simulink model "Arm_core_design_block"  (R2021a)
settings: Solver=VariableStepAuto  StartTime=0.0  StopTime=600  RelTol=1e-3
undefined symbols (not defined in the file or in its folder): AXI4, Lite
libraries: hdlBasic x979, xbsIndex_r4 x1
(part 1 of 7)
settings Model: Creator=jag33  LastModifiedBy=jag33

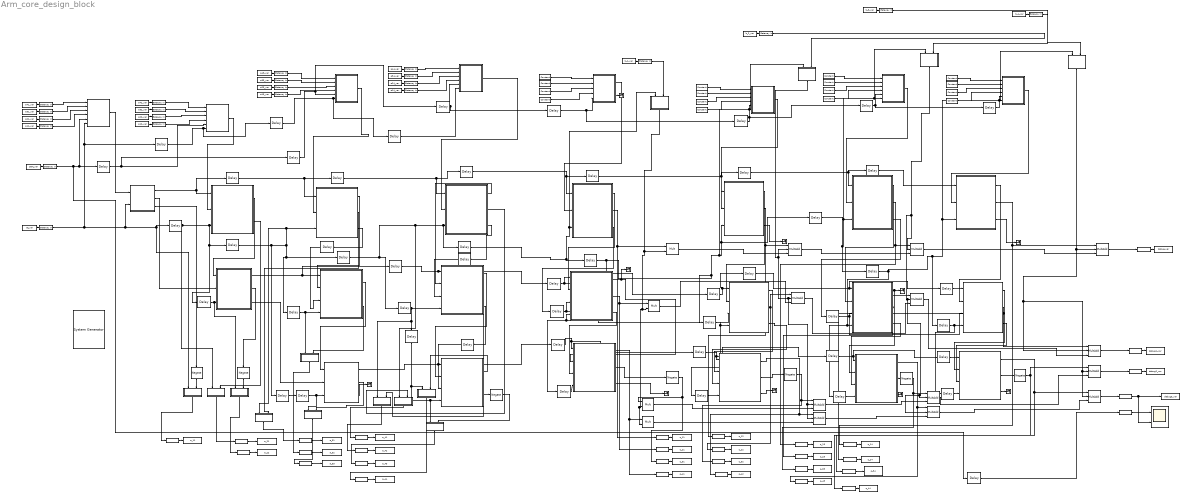
== system Arm_core_design_block ==
  " System Generator" : xbsIndex_r4/ System Generator  Tag=genX  xilinxfamily=zynq  part=xc7z020  speed=-1  package=clg484  synthesis_tool=Vivado  clock_wrapper=Clock Enables  directory=./../../../netlist_proj6_test6  proj_type=Vivado  Synth_file=Vivado Synthesis Defaults  Impl_file=Vivado Implementation Defaults  testbench=off  simulink_period=1  sysclk_period=10  dcm_input_clock_period=10  incr_netlist=off  trim_vbits=Everywhere in SubSystem  dbl_ovrd=According to Block Masks  core_generation=According to Block Masks  run_coregen=off  deprecated_control=off  eval_field=0  block_type=sysgen
  Constant{1..3,6..9,11..14,16} (12 alike) : hdlBasic/Constant  const=0  gui_display_data_type=Fixed-point  arith_type=Signed (2's comp)  n_bits=16  bin_pt=13  preci_type=Single  exp_width=8  frac_width=24  explicit_period=off  period=1  XmcBlockStatus=1  maskContainerNames=tabcontainer1  block_type=constant  block_config=sysgen:Constant_config
  Constant{4..5,10,15} (4 alike) : hdlBasic/Constant  const=1  gui_display_data_type=Fixed-point  arith_type=Signed (2's comp)  n_bits=16  bin_pt=13  preci_type=Single  exp_width=8  frac_width=24  explicit_period=off  period=1  XmcBlockStatus=1  maskContainerNames=tabcontainer1  block_type=constant  block_config=sysgen:Constant_config
  Delay : hdlBasic/Delay  rst=off  en=off  latency=330  reg_retiming=off  XmcBlockStatus=1  maskContainerNames=group1  block_type=delay  block_config=sysgen:Delay_config
  Delay{1..2,6,21,32} (5 alike) : hdlBasic/Delay  rst=off  en=off  latency=25  reg_retiming=off  XmcBlockStatus=1  maskContainerNames=group1  block_type=delay  block_config=sysgen:Delay_config
  Delay{3..5,7..20,22..31,33..49} (44 alike) : hdlBasic/Delay  rst=off  en=off  latency=24  reg_retiming=off  XmcBlockStatus=1  maskContainerNames=group1  block_type=delay  block_config=sysgen:Delay_config
  From Wor43pace1 : FromWorkspace  VariableName=a34_var
  From Work3pace19 : FromWorkspace  VariableName=a33_var
  From Workspace1 : FromWorkspace  VariableName=b_1_var
  From Workspace10 : FromWorkspace  VariableName=a11_var
  From Workspace11 : FromWorkspace  VariableName=a21_var
  From Workspace12 : FromWorkspace  VariableName=a31_var
  From Workspace13 : FromWorkspace  VariableName=a41_var
  From Workspace14 : FromWorkspace  VariableName=a12_var
  From Workspace15 : FromWorkspace  VariableName=a22_var
  From Workspace16 : FromWorkspace  VariableName=a32_var
  From Workspace17 : FromWorkspace  VariableName=a42_var
  From Workspace18 : FromWorkspace  VariableName=a23_var
  From Workspace19 : FromWorkspace  VariableName=a44_var
  From Workspace2 : FromWorkspace  VariableName=rst_var
  From Workspace20 : FromWorkspace  VariableName=a43_var
  From Workspace21 : FromWorkspace  VariableName=a14_var
  From Workspace3 : FromWorkspace  VariableName=start_var
  From Workspace4 : FromWorkspace  VariableName=a13_var
  From Workspace5 : FromWorkspace  VariableName=a24_var
  From Workspace6 : FromWorkspace  VariableName=b_2_var
  From Workspace7 : FromWorkspace  VariableName=b_3_var
  From Workspace8 : FromWorkspace  VariableName=b_4_var
  Mult : hdlBasic/Mult  precision=Full  arith_type="Signed  (2's comp)"  n_bits=16  bin_pt=13  quantization=Truncate  overflow=Wrap  en=off  latency=3  use_behavioral_HDL=off  opt=Speed  use_embedded=on  optimum_pipeline=off  pipeline=on  use_rpm=on  placement_style=Triangular  XmcBlockStatus=1  maskContainerNames=group1  block_type=mult  block_config=sysgen:Mult_config
  Mult1 : hdlBasic/Mult  precision=Full  arith_type="Signed  (2's comp)"  n_bits=16  bin_pt=13  quantization=Truncate  overflow=Wrap  en=off  latency=3  use_behavioral_HDL=off  opt=Speed  use_embedded=on  optimum_pipeline=off  pipeline=on  use_rpm=on  placement_style=Triangular  XmcBlockStatus=1  maskContainerNames=group1  block_type=mult  block_config=sysgen:Mult_config
  Mult2 : hdlBasic/Mult  precision=Full  arith_type="Signed  (2's comp)"  n_bits=16  bin_pt=13  quantization=Truncate  overflow=Wrap  en=off  latency=3  use_behavioral_HDL=off  opt=Speed  use_embedded=on  optimum_pipeline=off  pipeline=on  use_rpm=on  placement_style=Triangular  XmcBlockStatus=1  maskContainerNames=group1  block_type=mult  block_config=sysgen:Mult_config
  Mult3 : hdlBasic/Mult  precision=Full  arith_type="Signed  (2's comp)"  n_bits=16  bin_pt=14  quantization=Truncate  overflow=Wrap  en=off  latency=3  use_behavioral_HDL=off  opt=Speed  use_embedded=on  optimum_pipeline=off  pipeline=on  use_rpm=on  placement_style=Triangular  XmcBlockStatus=1  maskContainerNames=group1  block_type=mult  block_config=sysgen:Mult_config
  MultAdd : hdlBasic/MultAdd  mode=Addition  en=off  latency=0  precision=Full  arith_type="Signed  (2's comp)"  n_bits=16  bin_pt=13  XmcBlockStatus=1  maskContainerNames=tabcontainer1  block_type=multadd  block_config=sysgen:MultAdd_config
  MultAdd{1,7..10} (5 alike) : hdlBasic/MultAdd  mode=Addition  en=off  latency=0  precision=Full  arith_type=Unsigned  n_bits=16  bin_pt=14  XmcBlockStatus=1  maskContainerNames=tabcontainer1  block_type=multadd  block_config=sysgen:MultAdd_config
  MultAdd11 : hdlBasic/MultAdd  mode=Addition  en=off  latency=0  precision=User Defined  arith_type="Signed  (2's comp)"  n_bits=16  bin_pt=13  XmcBlockStatus=1  maskContainerNames=tabcontainer1  block_type=multadd  block_config=sysgen:MultAdd_config
  MultAdd2 : hdlBasic/MultAdd  mode=Addition  en=off  latency=0  precision=User Defined  arith_type="Signed  (2's comp)"  n_bits=16  bin_pt=13  XmcBlockStatus=1  maskContainerNames=tabcontainer1  block_type=multadd  block_config=sysgen:MultAdd_config
  MultAdd3 : hdlBasic/MultAdd  mode=Addition  en=off  latency=0  precision=Full  arith_type=Unsigned  n_bits=16  bin_pt=13  XmcBlockStatus=1  maskContainerNames=tabcontainer1  block_type=multadd  block_config=sysgen:MultAdd_config
  MultAdd4 : hdlBasic/MultAdd  mode=Addition  en=off  latency=0  precision=Full  arith_type=Unsigned  n_bits=16  bin_pt=13  XmcBlockStatus=1  maskContainerNames=tabcontainer1  block_type=multadd  block_config=sysgen:MultAdd_config
  MultAdd5 : hdlBasic/MultAdd  mode=Addition  en=off  latency=0  precision=User Defined  arith_type="Signed  (2's comp)"  n_bits=16  bin_pt=13  XmcBlockStatus=1  maskContainerNames=tabcontainer1  block_type=multadd  block_config=sysgen:MultAdd_config
  MultAdd6 : hdlBasic/MultAdd  mode=Addition  en=off  latency=0  precision=User Defined  arith_type=Unsigned  n_bits=16  bin_pt=13  XmcBlockStatus=1  maskContainerNames=tabcontainer1  block_type=multadd  block_config=sysgen:MultAdd_config
  Negate{1..4,6,8,10} (7 alike) : hdlBasic/Negate  precision=User Defined  arith_type="Signed  (2's comp)"  n_bits=16  bin_pt=13  quantization=Truncate  overflow=Wrap  en=off  latency=0  XmcBlockStatus=1  maskContainerNames=tabcontainer1  block_type=negate  block_config=sysgen:Negate_config
  Scope : Scope  NumInputPorts=2
  Subsystem : Subsystem
  Subsystem1 : Subsystem
  Subsystem10 : Subsystem
  Subsystem11 : Subsystem
  Subsystem13 : Subsystem
  Subsystem14 : Subsystem
  Subsystem15 : Subsystem
  Subsystem16 : Subsystem
  Subsystem17 : Subsystem
  Subsystem18 : Subsystem
  Subsystem19 : Subsystem
  Subsystem2 : Subsystem
  Subsystem20 : Subsystem
  Subsystem21 : Subsystem
  Subsystem22 : Subsystem
  Subsystem3 : Subsystem
  Subsystem4 : Subsystem
  Subsystem5 : Subsystem
  Subsystem6 : Subsystem
  Subsystem7 : Subsystem
  Subsystem8 : Subsystem
  Subsystem9 : Subsystem
  Terminator{,1..8,13} (10 alike) : Terminator
  To Workspace1 : ToWorkspace  VariableName=q_11  SaveFormat=Timeseries  SampleTime=-1
  To Workspace10 : ToWorkspace  VariableName=a_41  SaveFormat=Timeseries  SampleTime=-1
  To Workspace11 : ToWorkspace  VariableName=a_44  SaveFormat=Timeseries  SampleTime=-1
  To Workspace12 : ToWorkspace  VariableName=a_42  SaveFormat=Timeseries  SampleTime=-1
  To Workspace13 : ToWorkspace  VariableName=a_43  SaveFormat=Timeseries  SampleTime=-1
  To Workspace14 : ToWorkspace  VariableName=q_21  SaveFormat=Timeseries  SampleTime=-1
  To Workspace15 : ToWorkspace  VariableName=q_31  SaveFormat=Timeseries  SampleTime=-1
  To Workspace16 : ToWorkspace  VariableName=q_41  SaveFormat=Timeseries  SampleTime=-1
  To Workspace17 : ToWorkspace  VariableName=q_42  SaveFormat=Timeseries  SampleTime=-1
  To Workspace18 : ToWorkspace  VariableName=q_32  SaveFormat=Timeseries  SampleTime=-1
  To Workspace19 : ToWorkspace  VariableName=q_13  SaveFormat=Timeseries  SampleTime=-1
  To Workspace2 : ToWorkspace  VariableName=a_22  SaveFormat=Timeseries  SampleTime=-1
  To Workspace20 : ToWorkspace  VariableName=q_23  SaveFormat=Timeseries  SampleTime=-1
  To Workspace21 : ToWorkspace  VariableName=q_33  SaveFormat=Timeseries  SampleTime=-1
  To Workspace22 : ToWorkspace  VariableName=q_43  SaveFormat=Timeseries  SampleTime=-1
  To Workspace23 : ToWorkspace  VariableName=q_44  SaveFormat=Timeseries  SampleTime=-1
  To Workspace24 : ToWorkspace  VariableName=q_24  SaveFormat=Timeseries  SampleTime=-1
  To Workspace25 : ToWorkspace  VariableName=q_14  SaveFormat=Timeseries  SampleTime=-1
  To Workspace26 : ToWorkspace  VariableName=q_34  SaveFormat=Timeseries  SampleTime=-1
  To Workspace27 : ToWorkspace  VariableName=debug_var  SaveFormat=Timeseries  SampleTime=-1
  To Workspace28 : ToWorkspace  VariableName=debug1_var  SaveFormat=Timeseries  SampleTime=-1
  To Workspace29 : ToWorkspace  VariableName=debug2_var  SaveFormat=Timeseries  SampleTime=-1
  To Workspace3 : ToWorkspace  VariableName=a_11  SaveFormat=Timeseries  SampleTime=-1
  To Workspace30 : ToWorkspace  VariableName=debug3_var  SaveFormat=Timeseries  SampleTime=-1
  To Workspace4 : ToWorkspace  VariableName=q_12  SaveFormat=Timeseries  SampleTime=-1
  To Workspace5 : ToWorkspace  VariableName=a_21  SaveFormat=Timeseries  SampleTime=-1
  To Workspace6 : ToWorkspace  VariableName=a_31  SaveFormat=Timeseries  SampleTime=-1
  To Workspace7 : ToWorkspace  VariableName=q_22  SaveFormat=Timeseries  SampleTime=-1
  To Workspace8 : ToWorkspace  VariableName=a_32  SaveFormat=Timeseries  SampleTime=-1
  To Workspace9 : ToWorkspace  VariableName=a_33  SaveFormat=Timeseries  SampleTime=-1
  a11_var : hdlBasic/Gateway In  gui_display_data_type=Fixed-point  arith_type=Signed (2's comp)  n_bits=16  bin_pt=13  preci_type=Single  exp_width=8  frac_width=24  rows=1  columns=1  quantization="Round  (unbiased: +/- Inf)"  overflow=Saturate  period=1  UseAsADC=off  ADCChannel='1'  interface=AXI4-Lite  automatic_assignment=on  address_offset=hex2dec('00')  intf_name=''  intf_description=''  default_value=0  timing_constraint=None  locs_specified=off  LOCs={}  io_standard={}  inherit_from_input=off  hdl_port=on  XmcBlockStatus=1  maskContainerNames=group4  block_type=gatewayin  block_config=sysgen:gateway_in_config  block_width_w=590  block_height_w=620  block_width=640  block_height=850
  a12_var : hdlBasic/Gateway In  gui_display_data_type=Fixed-point  arith_type=Signed (2's comp)  n_bits=16  bin_pt=13  preci_type=Single  exp_width=8  frac_width=24  rows=1  columns=1  quantization="Round  (unbiased: +/- Inf)"  overflow=Saturate  period=1  UseAsADC=off  ADCChannel='1'  interface=AXI4-Lite  automatic_assignment=on  address_offset=hex2dec('00')  intf_name=''  intf_description=''  default_value=0  timing_constraint=None  locs_specified=off  LOCs={}  io_standard={}  inherit_from_input=off  hdl_port=on  XmcBlockStatus=1  maskContainerNames=group4  block_type=gatewayin  block_config=sysgen:gateway_in_config  block_width_w=590  block_height_w=620  block_width=640  block_height=850
  a13_var : hdlBasic/Gateway In  gui_display_data_type=Fixed-point  arith_type=Signed (2's comp)  n_bits=16  bin_pt=13  preci_type=Single  exp_width=8  frac_width=24  rows=1  columns=1  quantization="Round  (unbiased: +/- Inf)"  overflow=Saturate  period=1  UseAsADC=off  ADCChannel='1'  interface=AXI4-Lite  automatic_assignment=on  address_offset=hex2dec('00')  intf_name=''  intf_description=''  default_value=0  timing_constraint=None  locs_specified=off  LOCs={}  io_standard={}  inherit_from_input=off  hdl_port=on  XmcBlockStatus=1  maskContainerNames=group4  block_type=gatewayin  block_config=sysgen:gateway_in_config  block_width_w=590  block_height_w=620  block_width=640  block_height=850
  a14_var : hdlBasic/Gateway In  gui_display_data_type=Fixed-point  arith_type=Signed (2's comp)  n_bits=16  bin_pt=13  preci_type=Single  exp_width=8  frac_width=24  rows=1  columns=1  quantization="Round  (unbiased: +/- Inf)"  overflow=Saturate  period=1  UseAsADC=off  ADCChannel='1'  interface=AXI4-Lite  automatic_assignment=on  address_offset=hex2dec('00')  intf_name=''  intf_description=''  default_value=0  timing_constraint=None  locs_specified=off  LOCs={}  io_standard={}  inherit_from_input=off  hdl_port=on  XmcBlockStatus=1  maskContainerNames=group4  block_type=gatewayin  block_config=sysgen:gateway_in_config  block_width_w=590  block_height_w=620  block_width=640  block_height=850
  a21_var : hdlBasic/Gateway In  gui_display_data_type=Fixed-point  arith_type=Signed (2's comp)  n_bits=16  bin_pt=13  preci_type=Single  exp_width=8  frac_width=24  rows=1  columns=1  quantization="Round  (unbiased: +/- Inf)"  overflow=Saturate  period=1  UseAsADC=off  ADCChannel='1'  interface=AXI4-Lite  automatic_assignment=on  address_offset=hex2dec('00')  intf_name=''  intf_description=''  default_value=0  timing_constraint=None  locs_specified=off  LOCs={}  io_standard={}  inherit_from_input=off  hdl_port=on  XmcBlockStatus=1  maskContainerNames=group4  block_type=gatewayin  block_config=sysgen:gateway_in_config  block_width_w=590  block_height_w=620  block_width=640  block_height=850
  a22_var : hdlBasic/Gateway In  gui_display_data_type=Fixed-point  arith_type=Signed (2's comp)  n_bits=16  bin_pt=13  preci_type=Single  exp_width=8  frac_width=24  rows=1  columns=1  quantization="Round  (unbiased: +/- Inf)"  overflow=Saturate  period=1  UseAsADC=off  ADCChannel='1'  interface=AXI4-Lite  automatic_assignment=on  address_offset=hex2dec('00')  intf_name=''  intf_description=''  default_value=0  timing_constraint=None  locs_specified=off  LOCs={}  io_standard={}  inherit_from_input=off  hdl_port=on  XmcBlockStatus=1  maskContainerNames=group4  block_type=gatewayin  block_config=sysgen:gateway_in_config  block_width_w=590  block_height_w=620  block_width=640  block_height=850
  a23_var : hdlBasic/Gateway In  gui_display_data_type=Fixed-point  arith_type=Signed (2's comp)  n_bits=16  bin_pt=13  preci_type=Single  exp_width=8  frac_width=24  rows=1  columns=1  quantization="Round  (unbiased: +/- Inf)"  overflow=Saturate  period=1  UseAsADC=off  ADCChannel='1'  interface=AXI4-Lite  automatic_assignment=on  address_offset=hex2dec('00')  intf_name=''  intf_description=''  default_value=0  timing_constraint=None  locs_specified=off  LOCs={}  io_standard={}  inherit_from_input=off  hdl_port=on  XmcBlockStatus=1  maskContainerNames=group4  block_type=gatewayin  block_config=sysgen:gateway_in_config  block_width_w=590  block_height_w=620  block_width=640  block_height=850
  a24_var : hdlBasic/Gateway In  gui_display_data_type=Fixed-point  arith_type=Signed (2's comp)  n_bits=16  bin_pt=13  preci_type=Single  exp_width=8  frac_width=24  rows=1  columns=1  quantization="Round  (unbiased: +/- Inf)"  overflow=Saturate  period=1  UseAsADC=off  ADCChannel='1'  interface=AXI4-Lite  automatic_assignment=on  address_offset=hex2dec('00')  intf_name=''  intf_description=''  default_value=0  timing_constraint=None  locs_specified=off  LOCs={}  io_standard={}  inherit_from_input=off  hdl_port=on  XmcBlockStatus=1  maskContainerNames=group4  block_type=gatewayin  block_config=sysgen:gateway_in_config  block_width_w=590  block_height_w=620  block_width=640  block_height=850
  a31_var : hdlBasic/Gateway In  gui_display_data_type=Fixed-point  arith_type=Signed (2's comp)  n_bits=16  bin_pt=13  preci_type=Single  exp_width=8  frac_width=24  rows=1  columns=1  quantization="Round  (unbiased: +/- Inf)"  overflow=Saturate  period=1  UseAsADC=off  ADCChannel='1'  interface=AXI4-Lite  automatic_assignment=on  address_offset=hex2dec('00')  intf_name=''  intf_description=''  default_value=0  timing_constraint=None  locs_specified=off  LOCs={}  io_standard={}  inherit_from_input=off  hdl_port=on  XmcBlockStatus=1  maskContainerNames=group4  block_type=gatewayin  block_config=sysgen:gateway_in_config  block_width_w=590  block_height_w=620  block_width=640  block_height=850
  a32_var : hdlBasic/Gateway In  gui_display_data_type=Fixed-point  arith_type=Signed (2's comp)  n_bits=16  bin_pt=13  preci_type=Single  exp_width=8  frac_width=24  rows=1  columns=1  quantization="Round  (unbiased: +/- Inf)"  overflow=Saturate  period=1  UseAsADC=off  ADCChannel='1'  interface=AXI4-Lite  automatic_assignment=on  address_offset=hex2dec('00')  intf_name=''  intf_description=''  default_value=0  timing_constraint=None  locs_specified=off  LOCs={}  io_standard={}  inherit_from_input=off  hdl_port=on  XmcBlockStatus=1  maskContainerNames=group4  block_type=gatewayin  block_config=sysgen:gateway_in_config  block_width_w=590  block_height_w=620  block_width=640  block_height=850
  a33_var : hdlBasic/Gateway In  gui_display_data_type=Fixed-point  arith_type=Signed (2's comp)  n_bits=16  bin_pt=13  preci_type=Single  exp_width=8  frac_width=24  rows=1  columns=1  quantization="Round  (unbiased: +/- Inf)"  overflow=Saturate  period=1  UseAsADC=off  ADCChannel='1'  interface=AXI4-Lite  automatic_assignment=on  address_offset=hex2dec('00')  intf_name=''  intf_description=''  default_value=0  timing_constraint=None  locs_specified=off  LOCs={}  io_standard={}  inherit_from_input=off  hdl_port=on  XmcBlockStatus=1  maskContainerNames=group4  block_type=gatewayin  block_config=sysgen:gateway_in_config  block_width_w=590  block_height_w=620  block_width=640  block_height=850
  a34_var : hdlBasic/Gateway In  gui_display_data_type=Fixed-point  arith_type=Signed (2's comp)  n_bits=16  bin_pt=13  preci_type=Single  exp_width=8  frac_width=24  rows=1  columns=1  quantization="Round  (unbiased: +/- Inf)"  overflow=Saturate  period=1  UseAsADC=off  ADCChannel='1'  interface=AXI4-Lite  automatic_assignment=on  address_offset=hex2dec('00')  intf_name=''  intf_description=''  default_value=0  timing_constraint=None  locs_specified=off  LOCs={}  io_standard={}  inherit_from_input=off  hdl_port=on  XmcBlockStatus=1  maskContainerNames=group4  block_type=gatewayin  block_config=sysgen:gateway_in_config  block_width_w=590  block_height_w=620  block_width=640  block_height=850
  a41_var : hdlBasic/Gateway In  gui_display_data_type=Fixed-point  arith_type=Signed (2's comp)  n_bits=16  bin_pt=13  preci_type=Single  exp_width=8  frac_width=24  rows=1  columns=1  quantization="Round  (unbiased: +/- Inf)"  overflow=Saturate  period=1  UseAsADC=off  ADCChannel='1'  interface=AXI4-Lite  automatic_assignment=on  address_offset=hex2dec('00')  intf_name=''  intf_description=''  default_value=0  timing_constraint=None  locs_specified=off  LOCs={}  io_standard={}  inherit_from_input=off  hdl_port=on  XmcBlockStatus=1  maskContainerNames=group4  block_type=gatewayin  block_config=sysgen:gateway_in_config  block_width_w=590  block_height_w=620  block_width=640  block_height=850
  a42_var : hdlBasic/Gateway In  gui_display_data_type=Fixed-point  arith_type=Signed (2's comp)  n_bits=16  bin_pt=13  preci_type=Single  exp_width=8  frac_width=24  rows=1  columns=1  quantization="Round  (unbiased: +/- Inf)"  overflow=Saturate  period=1  UseAsADC=off  ADCChannel='1'  interface=AXI4-Lite  automatic_assignment=on  address_offset=hex2dec('00')  intf_name=''  intf_description=''  default_value=0  timing_constraint=None  locs_specified=off  LOCs={}  io_standard={}  inherit_from_input=off  hdl_port=on  XmcBlockStatus=1  maskContainerNames=group4  block_type=gatewayin  block_config=sysgen:gateway_in_config  block_width_w=590  block_height_w=620  block_width=640  block_height=850
  a43_var : hdlBasic/Gateway In  gui_display_data_type=Fixed-point  arith_type=Signed (2's comp)  n_bits=16  bin_pt=13  preci_type=Single  exp_width=8  frac_width=24  rows=1  columns=1  quantization="Round  (unbiased: +/- Inf)"  overflow=Saturate  period=1  UseAsADC=off  ADCChannel='1'  interface=AXI4-Lite  automatic_assignment=on  address_offset=hex2dec('00')  intf_name=''  intf_description=''  default_value=0  timing_constraint=None  locs_specified=off  LOCs={}  io_standard={}  inherit_from_input=off  hdl_port=on  XmcBlockStatus=1  maskContainerNames=group4  block_type=gatewayin  block_config=sysgen:gateway_in_config  block_width_w=590  block_height_w=620  block_width=640  block_height=850
  a44_var : hdlBasic/Gateway In  gui_display_data_type=Fixed-point  arith_type=Signed (2's comp)  n_bits=16  bin_pt=13  preci_type=Single  exp_width=8  frac_width=24  rows=1  columns=1  quantization="Round  (unbiased: +/- Inf)"  overflow=Saturate  period=1  UseAsADC=off  ADCChannel='1'  interface=AXI4-Lite  automatic_assignment=on  address_offset=hex2dec('00')  intf_name=''  intf_description=''  default_value=0  timing_constraint=None  locs_specified=off  LOCs={}  io_standard={}  inherit_from_input=off  hdl_port=on  XmcBlockStatus=1  maskContainerNames=group4  block_type=gatewayin  block_config=sysgen:gateway_in_config  block_width_w=590  block_height_w=620  block_width=640  block_height=850
  arctan1 : Subsystem
  arctan2 : Subsystem
  arctan3 : Subsystem
  b_{1..4} (4 alike) : hdlBasic/Gateway In  gui_display_data_type=Fixed-point  arith_type=Signed (2's comp)  n_bits=16  bin_pt=13  preci_type=Single  exp_width=8  frac_width=24  rows=1  columns=1  quantization="Round  (unbiased: +/- Inf)"  overflow=Saturate  period=1  UseAsADC=off  ADCChannel='1'  interface=AXI4-Lite  automatic_assignment=on  address_offset=hex2dec('00')  intf_name=''  intf_description=''  default_value=0  timing_constraint=None  locs_specified=off  LOCs={}  io_standard={}  inherit_from_input=off  hdl_port=on  XmcBlockStatus=1  maskContainerNames=group4  block_type=gatewayin  block_config=sysgen:gateway_in_config  block_width_w=590  block_height_w=620  block_width=640  block_height=850
  done_var : hdlBasic/Gateway Out  inherit_from_input=off  hdl_port=on  rows=1  columns=1  UseAsDAC=off  DACChannel='1'  interface=AXI4-Lite  automatic_assignment=on  address_offset=hex2dec('00')  intf_name=''  intf_description=''  timing_constraint=None  locs_specified=off  LOCs={}  io_standard={}  XmcBlockStatus=1  maskContainerNames=group4  block_type=gatewayout  block_config=sysgen:gateway_out_config  block_width_w=590  block_height_w=620  block_width=620  block_height=750
  qout_{1..4,11..14,21..24,31..34,41..44} (20 alike) : hdlBasic/Gateway Out  inherit_from_input=off  hdl_port=on  rows=1  columns=1  UseAsDAC=off  DACChannel='1'  interface=AXI4-Lite  automatic_assignment=on  address_offset=hex2dec('00')  intf_name=''  intf_description=''  timing_constraint=None  locs_specified=off  LOCs={}  io_standard={}  XmcBlockStatus=1  maskContainerNames=group4  block_type=gatewayout  block_config=sysgen:gateway_out_config  block_width_w=590  block_height_w=620  block_width=620  block_height=750
  rotation1 : Subsystem
  rotation10 : Subsystem
  rotation11 : Subsystem
  rotation12 : Subsystem
  rotation13 : Subsystem
  rotation14 : Subsystem
  rotation15 : Subsystem
  rotation16 : Subsystem
  rotation17 : Subsystem
  rotation19 : Subsystem
  rotation2 : Subsystem
  rotation3 : Subsystem
  rotation4 : Subsystem
  rotation5 : Subsystem
  rotation6 : Subsystem
  rotation7 : Subsystem
  rotation8 : Subsystem
  rotation9 : Subsystem
  rout_{11,21..22,31..33,41..44} (10 alike) : hdlBasic/Gateway Out  inherit_from_input=off  hdl_port=on  rows=1  columns=1  UseAsDAC=off  DACChannel='1'  interface=AXI4-Lite  automatic_assignment=on  address_offset=hex2dec('00')  intf_name=''  intf_description=''  timing_constraint=None  locs_specified=off  LOCs={}  io_standard={}  XmcBlockStatus=1  maskContainerNames=group4  block_type=gatewayout  block_config=sysgen:gateway_out_config  block_width_w=590  block_height_w=620  block_width=620  block_height=750
  rst_var : hdlBasic/Gateway In  gui_display_data_type=Boolean  arith_type=Boolean  n_bits=16  bin_pt=13  preci_type=Single  exp_width=8  frac_width=24  rows=1  columns=1  quantization="Round  (unbiased: +/- Inf)"  overflow=Saturate  period=1  UseAsADC=off  ADCChannel='1'  interface=AXI4-Lite  automatic_assignment=on  address_offset=hex2dec('00')  intf_name=''  intf_description=''  default_value=0  timing_constraint=None  locs_specified=off  LOCs={}  io_standard={}  inherit_from_input=off  hdl_port=on  XmcBlockStatus=1  maskContainerNames=group4  block_type=gatewayin  block_config=sysgen:gateway_in_config  block_width_w=590  block_height_w=620  block_width=640  block_height=850
  start_var : hdlBasic/Gateway In  gui_display_data_type=Boolean  arith_type=Boolean  n_bits=16  bin_pt=13  preci_type=Single  exp_width=8  frac_width=24  rows=1  columns=1  quantization="Round  (unbiased: +/- Inf)"  overflow=Saturate  period=1  UseAsADC=off  ADCChannel='1'  interface=AXI4-Lite  automatic_assignment=on  address_offset=hex2dec('00')  intf_name=''  intf_description=''  default_value=0  timing_constraint=None  locs_specified=off  LOCs={}  io_standard={}  inherit_from_input=off  hdl_port=on  XmcBlockStatus=1  maskContainerNames=group4  block_type=gatewayin  block_config=sysgen:gateway_in_config  block_width_w=590  block_height_w=620  block_width=640  block_height=850
  wires:
  Subsystem14/1(fifo_out) -> rotation1/2(y_in)
  rotation1/1(s_out) -> arctan2/1(y_in)
  rout_21/1 -> To Workspace5/1  "rout_21"
  rout_11/1 -> To Workspace3/1  "c"
  rotation1/2(c_out1) -> Subsystem1/2(reg_i)
  arctan1/1(out_theta) -> Delay5/1, rotation1/1(Theta_in)
  rout_31/1 -> To Workspace6/1  "out_31"
  rotation2/1(s_out) -> rotation3/2(y_in)
  Subsystem21/1(fifo_out) -> rotation2/2(y_in)
  rout_22/1 -> To Workspace2/1  "out_22"
  arctan1/2(ready) -> arctan2/2(sel)
  arctan2/1(out_theta) -> rotation3/1(Theta_in), Delay4/1
  rotation2/3(sel_out) -> Delay2/1
  Delay2/1 -> rotation3/3(sel_in)
  Delay5/1 -> rotation2/1(Theta_in), Delay3/1
  Delay3/1 -> rotation4/1(Theta_in), Delay7/1
  Subsystem11/1(fifo_out) -> rotation4/2(y_in)
  rotation2/2(c_out1) -> Subsystem3/2(reg_i)
  rout_32/1 -> To Workspace8/1  "out_32"
  arctan2/3(ready) -> arctan3/2(sel)
  rout_33/1 -> To Workspace9/1  "out_33"
  arctan2/2(cos_val) -> Negate3/1
  arctan3/3(ready) -> Terminator/1
  arctan3/1(out_theta) -> Delay22/1, rotation6/1(Theta_in)
  rotation4/3(sel_out) -> Delay1/1
  rotation4/1(s_out) -> rotation5/2(y_in)
  rotation3/1(s_out) -> arctan3/1(y_in)
  rotation3/2(c_out1) -> Subsystem4/2(reg_i)
  rout_41/1 -> To Workspace10/1  "out_41"
  Delay1/1 -> rotation5/3(sel_in)
  Delay4/1 -> Delay20/1, rotation5/1(Theta_in)
  rout_42/1 -> To Workspace12/1  "out_42"
  rotation5/2(c_out1) -> Subsystem7/2(reg_i)
  rotation5/1(s_out) -> rotation6/2(y_in)
  rotation5/3(sel_out) -> Delay6/1
  Delay6/1 -> rotation6/3(sel_in)
  rout_44/1 -> To Workspace11/1  "out_44"
  rout_43/1 -> To Workspace13/1  "out_43"
  Negate2/1 -> Subsystem8/2(reg_i)
  rotation6/2(c_out1) -> Negate2/1
  Subsystem13/1(fifo_out) -> rotation8/2(y_in)
  Delay7/1 -> rotation8/1(Theta_in), Delay19/1
  rotation8/3(sel_out) -> Delay21/1
  qout_11/1 -> To Workspace1/1  "c_r_out"
  rotation8/2(c_out1) -> qout_11/1, Mult/1
  From Workspace2/1 -> rst_var/1
  Delay8/1 -> Delay9/1, Delay12/1, rotation1/3(rst), Subsystem1/1(rst)
  Delay9/1 -> Delay13/1, Delay10/1, rotation2/3(rst), Subsystem3/1(rst), Delay14/1
  Delay12/1 -> Subsystem2/1(rst), arctan2/3(rst)
  Delay13/1 -> Subsystem4/1(rst), rotation3/4(rst)
  Delay14/1 -> Delay15/1
  Delay15/1 -> Subsystem5/1(rst), arctan3/3(rst)
  Delay16/1 -> Subsystem7/1(rst), Delay17/1, rotation5/4(rst)
  Delay17/1 -> Subsystem9/1(rst), rotation6/4(rst), Subsystem8/1(rst)
  Subsystem16/1(fifo_out) -> rotation7/2(y_in)
  Delay19/1 -> rotation7/1(Theta_in), Delay40/1
  rotation7/2(c_out1) -> qout_12/1, MultAdd/1
  rotation7/3(sel_out) -> Terminator4/1
  qout_12/1 -> To Workspace4/1  "c_r_out"
  qout_22/1 -> To Workspace7/1  "c_r_out"
  Delay20/1 -> Delay25/1, rotation9/1(Theta_in)
  rotation8/1(s_out) -> rotation9/2(y_in)
  Delay21/1 -> rotation11/3(sel_in), rotation9/3(sel_in)
  qout_21/1 -> To Workspace14/1  "c_r_out"
  rotation9/2(c_out1) -> qout_21/1, Mult1/1
  rotation9/1(s_out) -> rotation10/2(y_in), Terminator2/1
  rotation9/3(sel_out) -> rotation10/3(sel_in)
  Delay22/1 -> rotation10/1(Theta_in), Delay27/1
  Delay23/1 -> rotation10/4(rst)
  qout_31/1 -> To Workspace15/1  "c_r_out"
  rotation10/2(c_out1) -> Negate4/1
  rotation10/3(sel_out) -> Terminator3/1
  Delay18/1 -> Subsystem22/1(rst), Subsystem16/6(rst), rotation7/3(rst), Delay44/1, Delay26/1, Delay23/1, rotation9/4(rst)
  qout_41/1 -> To Workspace16/1  "c_r_out"
  Negate4/1 -> qout_31/1, Mult2/1
  rotation10/1(s_out) -> Mult3/1, qout_41/1
  rotation7/1(s_out) -> rotation11/2(y_in)
  Delay25/1 -> Delay41/1, rotation11/1(Theta_in)
  Delay26/1 -> rotation11/4(rst), Delay28/1
  rotation11/2(c_out1) -> qout_22/1, MultAdd3/1
  rotation11/1(s_out) -> rotation12/2(y_in)
  rotation11/3(sel_out) -> rotation12/3(sel_in)
  qout_42/1 -> To Workspace17/1  "c_r_out"
  qout_32/1 -> To Workspace18/1  "c_r_out"
  rotation12/2(c_out1) -> Negate6/1
  rotation12/1(s_out) -> MultAdd10/1, qout_42/1
  Delay28/1 -> rotation12/4(rst)
  rotation12/3(sel_out) -> Terminator5/1
  Delay27/1 -> rotation12/1(Theta_in), Delay33/1
  Subsystem15/1(fifo_out) -> rotation19/2(y_in)
  qout_24/1 -> To Workspace24/1  "c_r_out"
  Delay39/1 -> rotation15/4(rst)
  rotation16/3(sel_out) -> Terminator7/1
  Delay32/1 -> rotation14/3(sel_in), rotation17/3(sel_in)
  rotation19/1(s_out) -> rotation17/2(y_in)
  rotation16/1(s_out) -> rotation14/2(y_in)
  Delay44/1 -> Subsystem19/1(rst), Subsystem15/6(rst), rotation19/3(rst), Delay29/1
  qout_44/1 -> To Workspace23/1  "c_r_out"
  rotation17/3(sel_out) -> rotation13/3(sel_in)
  rotation19/2(c_out1) -> qout_13/1, MultAdd1/1
  Delay38/1 -> rotation15/1(Theta_in)
  Delay40/1 -> Delay30/1, rotation19/1(Theta_in)
  Delay41/1 -> rotation17/1(Theta_in), Delay36/1
  Negate8/1 -> MultAdd7/1, qout_33/1
  qout_13/1 -> To Workspace19/1  "c_r_out"
  qout_14/1 -> To Workspace25/1  "c_r_out"
  qout_23/1 -> To Workspace20/1  "c_r_out"
  rotation16/2(c_out1) -> qout_14/1, MultAdd2/1
  rotation15/1(s_out) -> qout_44/1, MultAdd11/1
  Delay36/1 -> rotation14/1(Theta_in)
  rotation14/2(c_out1) -> MultAdd5/1, qout_24/1
  rotation15/2(c_out1) -> Negate10/1
  rotation19/3(sel_out) -> Delay32/1
  qout_33/1 -> To Workspace21/1  "c_r_out"
  qout_43/1 -> To Workspace22/1  "c_r_out"
  rotation15/3(sel_out) -> Terminator8/1
  qout_34/1 -> To Workspace26/1  "c_r_out"
  rotation13/2(c_out1) -> Negate8/1
  Delay29/1 -> rotation16/3(rst), Subsystem20/1(rst), Subsystem17/6(rst), Delay37/1, rotation17/4(rst), Delay34/1
  Delay33/1 -> rotation13/1(Theta_in), Delay38/1
  rotation13/1(s_out) -> MultAdd8/1, qout_43/1
  rotation14/1(s_out) -> rotation15/2(y_in)
  rotation13/3(sel_out) -> Terminator6/1
  Delay30/1 -> rotation16/1(Theta_in)
  rotation17/1(s_out) -> rotation13/2(y_in), Terminator1/1
  rotation17/2(c_out1) -> MultAdd4/1, qout_23/1
  Subsystem17/1(fifo_out) -> rotation16/2(y_in)
  Delay37/1 -> rotation14/4(rst), Delay39/1
  Delay34/1 -> rotation13/4(rst)
  rotation14/3(sel_out) -> rotation15/3(sel_in)
  Negate10/1 -> MultAdd6/1, qout_34/1
  rotation6/1(s_out) -> Subsystem9/2(reg_i)
  arctan1/3(out) -> Negate1/1
  rotation4/2(c_out1) -> Subsystem6/2(reg_i)  "c_r_out"
  Subsystem/1(reg_o) -> rout_11/1
  Subsystem1/1(reg_o) -> rout_21/1
  Subsystem2/1(reg_o) -> rout_22/1
  Negate3/1 -> Subsystem2/2(reg_i)
  Subsystem3/1(reg_o) -> rout_31/1
  Subsystem4/1(reg_o) -> rout_32/1
  Subsystem5/1(reg_o) -> rout_33/1
  arctan3/2(cos_val) -> Subsystem5/2(reg_i)
  Negate1/1 -> Subsystem/2(reg_i)
  Subsystem8/1(reg_o) -> rout_43/1
  Subsystem6/1(reg_o) -> rout_41/1
  Subsystem7/1(reg_o) -> rout_42/1
  Subsystem9/1(reg_o) -> rout_44/1
  a41_var/1 -> Subsystem10/1(a4i)
  From Workspace10/1 -> a11_var/1
  From Workspace13/1 -> a41_var/1
  a21_var/1 -> Subsystem10/3(a2i)
  a11_var/1 -> Subsystem10/4(a1i)
  From Workspace11/1 -> a21_var/1
  From Workspace12/1 -> a31_var/1
  a31_var/1 -> Subsystem10/2(a3i)
  Subsystem10/1(fifo_out) -> arctan1/1(y_in)
  From Workspace3/1 -> start_var/1
  a32_var/1 -> Subsystem14/2(a3i)
  From Workspace16/1 -> a32_var/1
  From Workspace14/1 -> a12_var/1
  a22_var/1 -> Subsystem14/3(a2i)
  a12_var/1 -> Subsystem14/4(a1i)
  From Workspace15/1 -> a22_var/1
  a42_var/1 -> Subsystem14/1(a4i)
  From Workspace17/1 -> a42_var/1
  Delay24/1 -> Subsystem14/5(start), Delay31/1
  Delay31/1 -> Subsystem21/5(start), Delay35/1
  rst_var/1 -> Delay47/1, Subsystem10/6(rst), Delay8/1, Subsystem/1(rst), arctan1/2(rst)
  From Workspace20/1 -> a43_var/1
  a13_var/1 -> Subsystem21/4(a1i)
  a43_var/1 -> Subsystem21/1(a4i)
  From Work3pace19/1 -> a33_var/1
  a23_var/1 -> Subsystem21/3(a2i)
  From Workspace18/1 -> a23_var/1
  From Workspace4/1 -> a13_var/1
  a33_var/1 -> Subsystem21/2(a3i)
  a14_var/1 -> Subsystem11/4(a1i)
  From Wor43pace1/1 -> a34_var/1
  From Workspace5/1 -> a24_var/1
  a24_var/1 -> Subsystem11/3(a2i)
  From Workspace21/1 -> a14_var/1
  a34_var/1 -> Subsystem11/2(a3i)
  From Workspace19/1 -> a44_var/1
  Delay35/1 -> Delay42/1, Subsystem11/5(start)
  a44_var/1 -> Subsystem11/1(a4i)
  Delay10/1 -> Delay11/1, rotation4/3(rst), Subsystem6/1(rst), Delay16/1
  Delay42/1 -> Subsystem13/5(start), Delay45/1
  Constant3/1 -> Subsystem13/1(a4i)
  Constant1/1 -> Subsystem13/2(a3i)
  Constant4/1 -> Subsystem13/4(a1i)
  Constant2/1 -> Subsystem13/3(a2i)
  Delay11/1 -> Subsystem18/1(rst), rotation8/3(rst), Delay18/1
  Constant5/1 -> Subsystem15/2(a3i)
  Constant7/1 -> Subsystem15/1(a4i)
  Constant8/1 -> Subsystem15/4(a1i)
  Constant6/1 -> Subsystem15/3(a2i)
  Constant12/1 -> Subsystem16/4(a1i)
  Constant9/1 -> Subsystem16/2(a3i)
  Constant10/1 -> Subsystem16/3(a2i)
  Constant11/1 -> Subsystem16/1(a4i)
  Constant16/1 -> Subsystem17/4(a1i)
  Constant13/1 -> Subsystem17/2(a3i)
  Constant14/1 -> Subsystem17/3(a2i)
  Constant15/1 -> Subsystem17/1(a4i)
  Subsystem18/1(reg_o) -> Mult1/2, Mult2/2, Mult3/2, Mult/2
  From Workspace1/1 -> b_1/1
  b_1/1 -> Subsystem18/2(reg_i)
  Mult/1 -> MultAdd/3
  b_2/1 -> Subsystem22/2(reg_i)
  From Workspace6/1 -> b_2/1
  Delay45/1 -> Subsystem16/5(start), Delay43/1
  b_3/1 -> Subsystem19/2(reg_i)
  From Workspace7/1 -> b_3/1
  Delay43/1 -> Delay46/1, Subsystem15/5(start)
  b_4/1 -> Subsystem20/2(reg_i)
  From Workspace8/1 -> b_4/1
  Delay46/1 -> Subsystem17/5(start)
  MultAdd/1 -> MultAdd1/3
  Subsystem19/1(reg_o) -> MultAdd7/2, MultAdd8/2, MultAdd4/2, MultAdd1/2
  Subsystem22/1(reg_o) -> MultAdd9/2, MultAdd10/2, MultAdd3/2, MultAdd/2
  MultAdd1/1 -> MultAdd2/3
  Subsystem20/1(reg_o) -> MultAdd6/2, MultAdd11/2, MultAdd5/2, MultAdd2/2
  qout_1/1 -> To Workspace27/1  "c_r_out"
  Mult1/1 -> MultAdd3/3
  MultAdd3/1 -> MultAdd4/3
  MultAdd4/1 -> MultAdd5/3
  qout_2/1 -> To Workspace28/1  "c_r_out"
  MultAdd5/1 -> qout_2/1
  qout_3/1 -> To Workspace29/1  "c_r_out"
  MultAdd6/1 -> qout_3/1
  MultAdd9/1 -> MultAdd7/3
  MultAdd10/1 -> MultAdd8/3
  Mult3/1 -> MultAdd10/3
  Mult2/1 -> MultAdd9/3
  qout_4/1 -> To Workspace30/1, Scope/2  "c_r_out"
  MultAdd11/1 -> qout_4/1
  MultAdd7/1 -> MultAdd6/3
  MultAdd8/1 -> MultAdd11/3
  Negate6/1 -> MultAdd9/1, qout_32/1
  MultAdd2/1 -> qout_1/1
  Subsystem13/2(next_load) -> Terminator13/1
  Delay47/1 -> Delay48/1, Subsystem14/6(rst)
  Delay48/1 -> Delay49/1, Subsystem21/6(rst)
  Delay49/1 -> Subsystem11/6(rst)
  start_var/1 -> Subsystem10/5(start), Delay24/1, Delay/1
  Delay/1 -> done_var/1
  done_var/1 -> Scope/1  "c_r_out"

== system Arm_core_design_block/Subsystem ==
  rst : Inport
  reg_i : Inport  Port=2
  Absolute1 : hdlBasic/Absolute  precision=User Defined  arith_type="Signed  (2's comp)"  n_bits=16  bin_pt=13  quantization=Truncate  overflow=Saturate  en=off  latency=0  XmcBlockStatus=1  maskContainerNames=tabcontainer1  block_type=abs  block_config=sysgen:Abs_config
  Accumulator1 : hdlBasic/Accumulator  operation=Add  n_bits=16  overflow=Wrap  scale=1  rst=on  hasbypass=off  en=on  latency=1  msb_inp=100  msb=100  lsb=-100  use_behavioral_HDL=on  implementation=Fabric  XmcBlockStatus=1  maskContainerNames=group3  block_type=accum  block_config=sysgen:Accum_config
  Constant4 : hdlBasic/Constant  const=0.05  gui_display_data_type=Fixed-point  arith_type=Signed (2's comp)  n_bits=16  bin_pt=14  preci_type=Single  exp_width=8  frac_width=24  explicit_period=off  period=1  XmcBlockStatus=1  maskContainerNames=tabcontainer1  block_type=constant  block_config=sysgen:Constant_config
  Constant5 : hdlBasic/Constant  const=1  gui_display_data_type=Fixed-point  arith_type=Unsigned  n_bits=16  bin_pt=1  preci_type=Single  exp_width=8  frac_width=24  explicit_period=off  period=1  XmcBlockStatus=1  maskContainerNames=tabcontainer1  block_type=constant  block_config=sysgen:Constant_config
  Constant6 : hdlBasic/Constant  const=3  gui_display_data_type=Fixed-point  arith_type=Unsigned  n_bits=16  bin_pt=1  preci_type=Single  exp_width=8  frac_width=24  explicit_period=off  period=1  XmcBlockStatus=1  maskContainerNames=tabcontainer1  block_type=constant  block_config=sysgen:Constant_config
  Constant7 : hdlBasic/Constant  const=0  gui_display_data_type=Boolean  arith_type=Boolean  n_bits=16  bin_pt=1  preci_type=Single  exp_width=8  frac_width=24  explicit_period=off  period=1  XmcBlockStatus=1  maskContainerNames=tabcontainer1  block_type=constant  block_config=sysgen:Constant_config
  Mux1 : hdlBasic/Mux  inputs=2  en=off  latency=0  precision=Full  arith_type=Unsigned  n_bits=16  bin_pt=14  quantization=Truncate  overflow=Wrap  XmcBlockStatus=1  maskContainerNames=tabcontainer1  block_type=mux  block_config=sysgen:Mux_config
  Register1 : hdlBasic/Register  init=0  rst=on  en=on  XmcBlockStatus=1  maskContainerNames=tabcontainer1  block_type=register  block_config=sysgen:Register_config
  Relational2 : hdlBasic/Relational  mode=a>b  op_type=Bool  en=off  latency=0  XmcBlockStatus=1  maskContainerNames=tabcontainer1  block_type=relational  block_config=sysgen:Relational_config
  Relational3 : hdlBasic/Relational  mode=a>b  op_type=Bool  en=off  latency=0  XmcBlockStatus=1  maskContainerNames=tabcontainer1  block_type=relational  block_config=sysgen:Relational_config
  reg_o : Outport
  wires:
  Constant5/1 -> Accumulator1/1
  Relational2/1 -> Mux1/2
  Constant7/1 -> Mux1/3
  reg_i/1 -> Absolute1/1, Register1/1
  rst/1 -> Register1/2, Accumulator1/2
  Constant6/1 -> Relational3/2
  Accumulator1/1 -> Relational3/1
  Relational3/1 -> Mux1/1
  Mux1/1 -> Register1/3, Accumulator1/3
  Absolute1/1 -> Relational2/1
  Constant4/1 -> Relational2/2
  Register1/1 -> reg_o/1

== system Arm_core_design_block/Subsystem1 ==
  rst : Inport
  reg_i : Inport  Port=2
  Absolute1 : hdlBasic/Absolute  precision=User Defined  arith_type="Signed  (2's comp)"  n_bits=16  bin_pt=13  quantization=Truncate  overflow=Saturate  en=off  latency=0  XmcBlockStatus=1  maskContainerNames=tabcontainer1  block_type=abs  block_config=sysgen:Abs_config
  Accumulator1 : hdlBasic/Accumulator  operation=Add  n_bits=16  overflow=Wrap  scale=1  rst=on  hasbypass=off  en=on  latency=1  msb_inp=100  msb=100  lsb=-100  use_behavioral_HDL=on  implementation=Fabric  XmcBlockStatus=1  maskContainerNames=group3  block_type=accum  block_config=sysgen:Accum_config
  Constant4 : hdlBasic/Constant  const=0.05  gui_display_data_type=Fixed-point  arith_type=Signed (2's comp)  n_bits=16  bin_pt=14  preci_type=Single  exp_width=8  frac_width=24  explicit_period=off  period=1  XmcBlockStatus=1  maskContainerNames=tabcontainer1  block_type=constant  block_config=sysgen:Constant_config
  Constant5 : hdlBasic/Constant  const=1  gui_display_data_type=Fixed-point  arith_type=Unsigned  n_bits=16  bin_pt=1  preci_type=Single  exp_width=8  frac_width=24  explicit_period=off  period=1  XmcBlockStatus=1  maskContainerNames=tabcontainer1  block_type=constant  block_config=sysgen:Constant_config
  Constant6 : hdlBasic/Constant  const=3  gui_display_data_type=Fixed-point  arith_type=Unsigned  n_bits=16  bin_pt=1  preci_type=Single  exp_width=8  frac_width=24  explicit_period=off  period=1  XmcBlockStatus=1  maskContainerNames=tabcontainer1  block_type=constant  block_config=sysgen:Constant_config
  Constant7 : hdlBasic/Constant  const=0  gui_display_data_type=Boolean  arith_type=Boolean  n_bits=16  bin_pt=1  preci_type=Single  exp_width=8  frac_width=24  explicit_period=off  period=1  XmcBlockStatus=1  maskContainerNames=tabcontainer1  block_type=constant  block_config=sysgen:Constant_config
  Mux1 : hdlBasic/Mux  inputs=2  en=off  latency=0  precision=Full  arith_type=Unsigned  n_bits=16  bin_pt=14  quantization=Truncate  overflow=Wrap  XmcBlockStatus=1  maskContainerNames=tabcontainer1  block_type=mux  block_config=sysgen:Mux_config
  Register1 : hdlBasic/Register  init=0  rst=on  en=on  XmcBlockStatus=1  maskContainerNames=tabcontainer1  block_type=register  block_config=sysgen:Register_config
  Relational2 : hdlBasic/Relational  mode=a>b  op_type=Bool  en=off  latency=0  XmcBlockStatus=1  maskContainerNames=tabcontainer1  block_type=relational  block_config=sysgen:Relational_config
  Relational3 : hdlBasic/Relational  mode=a>b  op_type=Bool  en=off  latency=0  XmcBlockStatus=1  maskContainerNames=tabcontainer1  block_type=relational  block_config=sysgen:Relational_config
  reg_o : Outport
  wires:
  Constant5/1 -> Accumulator1/1
  Relational2/1 -> Mux1/2
  Constant7/1 -> Mux1/3
  reg_i/1 -> Absolute1/1, Register1/1
  rst/1 -> Register1/2, Accumulator1/2
  Constant6/1 -> Relational3/2
  Accumulator1/1 -> Relational3/1
  Relational3/1 -> Mux1/1
  Mux1/1 -> Register1/3, Accumulator1/3
  Absolute1/1 -> Relational2/1
  Constant4/1 -> Relational2/2
  Register1/1 -> reg_o/1

== system Arm_core_design_block/Subsystem10 ==
  a4i : Inport
  a3i : Inport  Port=2
  a2i : Inport  Port=3
  a1i : Inport  Port=4
  start : Inport  Port=5
  rst : Inport  Port=6
  Constant : hdlBasic/Constant  const=0  gui_display_data_type=Fixed-point  arith_type=Signed (2's comp)  n_bits=16  bin_pt=13  preci_type=Single  exp_width=8  frac_width=24  explicit_period=off  period=1  XmcBlockStatus=1  maskContainerNames=tabcontainer1  block_type=constant  block_config=sysgen:Constant_config
  Mux : hdlBasic/Mux  inputs=5  en=off  latency=0  precision=Full  arith_type=Unsigned  n_bits=16  bin_pt=14  quantization=Truncate  overflow=Wrap  XmcBlockStatus=1  maskContainerNames=tabcontainer1  block_type=mux  block_config=sysgen:Mux_config
  Subsystem10 : Subsystem
  Subsystem11 : Subsystem
  Subsystem12 : Subsystem
  Subsystem13 : Subsystem
  Subsystem14 : Subsystem
  Subsystem3 : Subsystem
  fifo_out : Outport
  wires:
  Subsystem14/1(reg_o) -> Mux/6
  Subsystem11/1(reg_o) -> Mux/3
  start/1 -> Subsystem10/1(reg_i)
  Subsystem13/1(reg_o) -> Mux/5
  Mux/1 -> fifo_out/1
  Subsystem12/1(reg_o) -> Mux/4
  a2i/1 -> Subsystem12/2(reg_i)
  Subsystem3/1(reg_o) -> Mux/1
  Constant/1 -> Mux/2
  Subsystem10/1(reg_o) -> Subsystem3/2(in_pulse)
  a3i/1 -> Subsystem13/2(reg_i)
  a4i/1 -> Subsystem14/2(reg_i)
  a1i/1 -> Subsystem11/2(reg_i)
  rst/1 -> Subsystem14/1(rst), Subsystem13/1(rst), Subsystem12/1(rst), Subsystem11/1(rst), Subsystem3/1(rst)

== system Arm_core_design_block/Subsystem11 ==
  a4i : Inport
  a3i : Inport  Port=2
  a2i : Inport  Port=3
  a1i : Inport  Port=4
  start : Inport  Port=5
  rst : Inport  Port=6
  Constant : hdlBasic/Constant  const=0  gui_display_data_type=Fixed-point  arith_type=Signed (2's comp)  n_bits=16  bin_pt=13  preci_type=Single  exp_width=8  frac_width=24  explicit_period=off  period=1  XmcBlockStatus=1  maskContainerNames=tabcontainer1  block_type=constant  block_config=sysgen:Constant_config
  Mux : hdlBasic/Mux  inputs=5  en=off  latency=0  precision=Full  arith_type=Unsigned  n_bits=16  bin_pt=14  quantization=Truncate  overflow=Wrap  XmcBlockStatus=1  maskContainerNames=tabcontainer1  block_type=mux  block_config=sysgen:Mux_config
  Subsystem10 : Subsystem
  Subsystem11 : Subsystem
  Subsystem12 : Subsystem
  Subsystem13 : Subsystem
  Subsystem14 : Subsystem
  Subsystem3 : Subsystem
  Terminator : Terminator
  fifo_out : Outport
  wires:
  Subsystem14/1(reg_o) -> Mux/6
  Subsystem11/1(reg_o) -> Mux/3
  start/1 -> Subsystem10/1(reg_i)
  Subsystem13/1(reg_o) -> Mux/5
  Mux/1 -> fifo_out/1
  Subsystem12/1(reg_o) -> Mux/4
  a2i/1 -> Subsystem12/2(reg_i)
  Subsystem3/1(reg_o) -> Mux/1
  Constant/1 -> Mux/2
  Subsystem10/1(reg_o) -> Subsystem3/2(in_pulse)
  a3i/1 -> Subsystem13/2(reg_i)
  a4i/1 -> Subsystem14/2(reg_i)
  a1i/1 -> Subsystem11/2(reg_i)
  rst/1 -> Subsystem14/1(rst), Subsystem13/1(rst), Subsystem12/1(rst), Subsystem11/1(rst), Subsystem3/1(rst)
  Subsystem3/2(rst_out) -> Terminator/1

== system Arm_core_design_block/Subsystem13 ==
  a4i : Inport
  a3i : Inport  Port=2
  a2i : Inport  Port=3
  a1i : Inport  Port=4
  start : Inport  Port=5
  Constant : hdlBasic/Constant  const=0  gui_display_data_type=Fixed-point  arith_type=Signed (2's comp)  n_bits=16  bin_pt=13  preci_type=Single  exp_width=8  frac_width=24  explicit_period=off  period=1  XmcBlockStatus=1  maskContainerNames=tabcontainer1  block_type=constant  block_config=sysgen:Constant_config
  Delay : hdlBasic/Delay  rst=off  en=off  latency=3  reg_retiming=off  XmcBlockStatus=1  maskContainerNames=group1  block_type=delay  block_config=sysgen:Delay_config
  Mux : hdlBasic/Mux  inputs=5  en=off  latency=0  precision=Full  arith_type=Unsigned  n_bits=16  bin_pt=14  quantization=Truncate  overflow=Wrap  XmcBlockStatus=1  maskContainerNames=tabcontainer1  block_type=mux  block_config=sysgen:Mux_config
  Subsystem10 : Subsystem
  Subsystem11 : Subsystem
  Subsystem12 : Subsystem
  Subsystem13 : Subsystem
  Subsystem14 : Subsystem
  Subsystem3 : Subsystem
  fifo_out : Outport
  next_load : Outport  Port=2
  wires:
  Subsystem14/1(reg_o) -> Mux/6
  Subsystem11/1(reg_o) -> Mux/3
  start/1 -> Subsystem10/1(reg_i)
  Subsystem13/1(reg_o) -> Mux/5
  Mux/1 -> fifo_out/1
  Subsystem12/1(reg_o) -> Mux/4
  a2i/1 -> Subsystem12/2(reg_i)
  Subsystem3/1(reg_o) -> Mux/1
  Constant/1 -> Mux/2
  Subsystem10/1(reg_o) -> Subsystem3/2(in_pulse)
  a3i/1 -> Subsystem13/2(reg_i)
  a4i/1 -> Subsystem14/2(reg_i)
  a1i/1 -> Subsystem11/2(reg_i)
  Delay/1 -> Subsystem14/1(rst), Subsystem13/1(rst), Subsystem12/1(rst), Subsystem11/1(rst), Subsystem3/1(rst)
  Subsystem3/2(rst_out) -> Delay/1, next_load/1

== system Arm_core_design_block/Subsystem14 ==
  a4i : Inport
  a3i : Inport  Port=2
  a2i : Inport  Port=3
  a1i : Inport  Port=4
  start : Inport  Port=5
  rst : Inport  Port=6
  Constant : hdlBasic/Constant  const=0  gui_display_data_type=Fixed-point  arith_type=Signed (2's comp)  n_bits=16  bin_pt=13  preci_type=Single  exp_width=8  frac_width=24  explicit_period=off  period=1  XmcBlockStatus=1  maskContainerNames=tabcontainer1  block_type=constant  block_config=sysgen:Constant_config
  Mux : hdlBasic/Mux  inputs=5  en=off  latency=0  precision=Full  arith_type=Unsigned  n_bits=16  bin_pt=14  quantization=Truncate  overflow=Wrap  XmcBlockStatus=1  maskContainerNames=tabcontainer1  block_type=mux  block_config=sysgen:Mux_config
  Subsystem10 : Subsystem
  Subsystem11 : Subsystem
  Subsystem12 : Subsystem
  Subsystem13 : Subsystem
  Subsystem14 : Subsystem
  Subsystem3 : Subsystem
  Terminator : Terminator
  fifo_out : Outport
  wires:
  Subsystem14/1(reg_o) -> Mux/6
  Subsystem11/1(reg_o) -> Mux/3
  start/1 -> Subsystem10/1(reg_i)
  Subsystem13/1(reg_o) -> Mux/5
  Mux/1 -> fifo_out/1
  Subsystem12/1(reg_o) -> Mux/4
  a2i/1 -> Subsystem12/2(reg_i)
  Subsystem3/1(reg_o) -> Mux/1
  Constant/1 -> Mux/2
  Subsystem10/1(reg_o) -> Subsystem3/2(in_pulse)
  a3i/1 -> Subsystem13/2(reg_i)
  a4i/1 -> Subsystem14/2(reg_i)
  a1i/1 -> Subsystem11/2(reg_i)
  rst/1 -> Subsystem14/1(rst), Subsystem13/1(rst), Subsystem12/1(rst), Subsystem11/1(rst), Subsystem3/1(rst)
  Subsystem3/2(rst_out) -> Terminator/1
